simulink model "Comparator"  (R2015a)
settings: Solver=ode23t  StartTime=0.0  StopTime=10.0  RelTol=1e-10
libraries: fl_lib x29, nesl_utility x9, elec_lib x6, pe_lib x1, powerlib x1
settings Model: Creator=saifur  LastModifiedBy=saifur

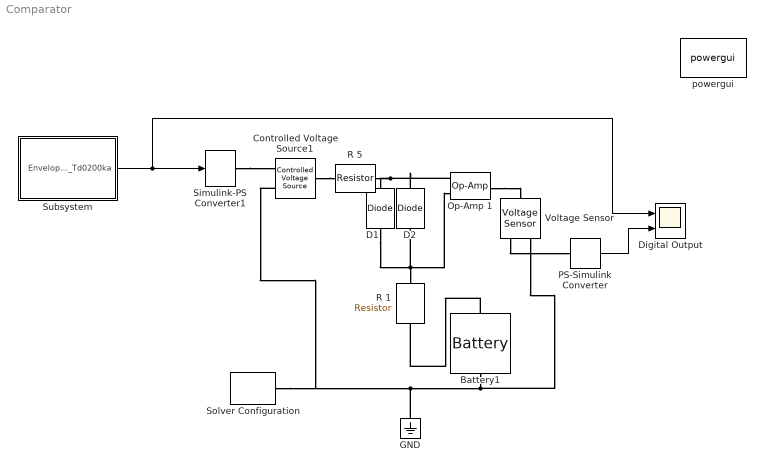
== system Comparator ==
  Battery1 : pe_lib/Sources/Battery  Vnom=6 V  AH=50 hr*A  AH0=50 hr*A  V1=0.5 V  AH1=25 hr*A  R1=2 Ohm  R2=inf Ohm  alpha=1  beta=1  G2=0 S
  Controlled Voltage Source1 : fl_lib/Electrical/Electrical Sources/Controlled Voltage Source
  D1 : fl_lib/Electrical/Electrical Elements/Diode  Vf=0.6 V  Ron=0.3 Ohm  Goff=1e-8 1/Ohm  i_specify=off  i_priority=High  i=0 A  v_specify=off  v_priority=High  v=0 V
  D2 : fl_lib/Electrical/Electrical Elements/Diode  Vf=0.6 V  Ron=0.3 Ohm  Goff=1e-8 1/Ohm  i_specify=off  i_priority=High  i=0 A  v_specify=off  v_priority=High  v=0 V
  Digital Output : Scope  NumInputPorts=2
      settings: TimeRange=10  YMin=-1~-1  YMax=1~1
  GND : fl_lib/Electrical/Electrical Elements/Electrical Reference
  Op-Amp 1 : fl_lib/Electrical/Electrical Elements/Op-Amp  outI_specify=off  outI_priority=High  outI=0 A
  PS-Simulink Converter : nesl_utility/PS-Simulink Converter  PhysicalDomain=network_engine_domain  SubClassName=ps_output  LeftPortType=input  RightPortType=output  PseudoPeriodic=off  Frequencies=[]  Unit=1  AffineConversion=off
  R 1 : elec_lib/Passive Devices/Resistor  R=2.154 kOhm  noise_mode=0  Tdevice=25 C  sample_time=0.001 s  repeatability=1  auto_seed=418932850  user_seed=0
  R 5 : elec_lib/Passive Devices/Resistor  R=2.5 kOhm  noise_mode=0  Tdevice=25 C  sample_time=0.001 s  repeatability=1  auto_seed=2715962282  user_seed=0
  Simulink-PS Converter1 : nesl_utility/Simulink-PS Converter  PhysicalDomain=network_engine_domain  SubClassName=ps_input  LeftPortType=input  RightPortType=output  PseudoPeriodic=off  Frequencies=[]  NoiseDistribution=none  NoiseParameters=[]  Unit=V  AffineConversion=off  InputFiltering=off  SimscapeFilterOrder=1  InputFilterTimeConstant=0.001  UdotUserProvided=1
  Solver Configuration : nesl_utility/Solver Configuration  PhysicalDomain=network_engine_domain  SubClassName=solver  LeftPortType=input  RightPortType=generic  Accelerate=off  Tones=[]  Harmonics=[]  SimulateNoise=off  Profile=off  UseLocalSampling=off  EnableSwitchedLinearOptims=on  FrequencyDomain=off  UseCCode=off  RelTol=0.001  AbsTol=1e-06  MinStep=1e-09  ToWorkspace=off  RevertToSquareIcSolve=off  NumHomotopyIterations=100  DoDC=on  ResidualTolerance=1e-09  UseLocalSolver=off  LocalSolverChoice=NE_BACKWARD_EULER_ADVANCER  LocalSolverSampleTime=0.001  DoFixedCost=off  MaxNonlinIter=3  MaxModeIter=2  LinearAlgebra=Sparse  DelaysMemoryBudget=1024  AutomaticFiltering=on  FilteringTimeConstant=0.001
  Subsystem : Subsystem
  Voltage Sensor : fl_lib/Electrical/Electrical Sensors/Voltage Sensor
  powergui : powerlib/powergui  Priority=1  SimulationMode=Continuous  SolverType=Tustin/Backward Euler (TBE)  SampleTime=50e-6  frequency=60  SPID=on  DisableSnubberDevices=off  DisableRonSwitches=off  DisableVfSwitches=off  SwTol=0  DisplayEquations=on  Interpol=off  methode=off  Ts=100  FunctionMessages=off  echomessages=off  HookPort=off  EnableUseOfTLC=off  x0status=blocks  frequencyindice=0  Pbase=100e6  ErrMax=1e-4  Iterations=50  UnitsV=kV  UnitsW=MW  buscounter=0  RestoreLinks=warning  ResistiveCurrentMeasurement=off  Frange=[0:2:500]  Ylog=off  Xlog=on  ShowGrid=off  save=off  variable=ZData  structure=0  ZoomFFT=off  StartTime=0.0  cycles=1  DisplayStyle=1  fundamental=60  FreqAxis=off  MaxFrequency=1000  frequencyindicesteady=1  RmsSteady=1  display=off
  wires:
  PS-Simulink Converter/1 -> Digital Output/2
  Subsystem/1("Envelope_Td0200ka ") -> Digital Output/1, Simulink-PS Converter1/1
  connections:
  Simulink-PS Converter1/RConn1 -- Controlled Voltage Source1/RConn1
  Controlled Voltage Source1/LConn1 -- R 5/RConn1
  Voltage Sensor/RConn1 -- PS-Simulink Converter/LConn1
  R 5/LConn1 -- Op-Amp 1/LConn1 -- D2/LConn1 -- D1/RConn1
  D1/LConn1 -- R 1/RConn1 -- D2/RConn1 -- Op-Amp 1/LConn2
  Battery1/LConn1 -- R 1/LConn1
  Controlled Voltage Source1/RConn2 -- Solver Configuration/RConn1 -- Voltage Sensor/RConn2 -- Battery1/RConn1 -- GND/LConn1
  Op-Amp 1/RConn1 -- Voltage Sensor/LConn1

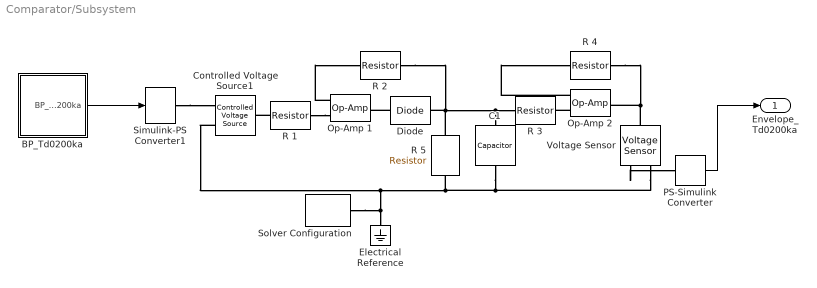
== system Comparator/Subsystem ==
  BP_Td0200ka : Subsystem
  C1 : fl_lib/Electrical/Electrical Elements/Capacitor  c=1e-6 F  r=1e-6 Ohm  g=0 1/Ohm  i_specify=off  i_priority=High  i=0 A  v_specify=off  v_priority=High  v=0 V  vc_specify=off  vc_priority=High  vc=0 V
  Controlled Voltage Source1 : fl_lib/Electrical/Electrical Sources/Controlled Voltage Source
  Diode : fl_lib/Electrical/Electrical Elements/Diode  Vf=0.6 V  Ron=0.3 Ohm  Goff=1e-8 1/Ohm  i_specify=off  i_priority=High  i=0 A  v_specify=off  v_priority=High  v=0 V
  Electrical Reference : fl_lib/Electrical/Electrical Elements/Electrical Reference
  Op-Amp 1 : fl_lib/Electrical/Electrical Elements/Op-Amp  outI_specify=off  outI_priority=High  outI=0 A
  Op-Amp 2 : fl_lib/Electrical/Electrical Elements/Op-Amp  outI_specify=off  outI_priority=High  outI=0 A
  PS-Simulink Converter : nesl_utility/PS-Simulink Converter  PhysicalDomain=network_engine_domain  SubClassName=ps_output  LeftPortType=input  RightPortType=output  PseudoPeriodic=off  Frequencies=[]  Unit=1  AffineConversion=off
  R 1 : fl_lib/Electrical/Electrical Elements/Resistor  R=1 Ohm  i_specify=off  i_priority=High  i=0 A  v_specify=off  v_priority=High  v=0 V
  R 2 : elec_lib/Passive Devices/Resistor  R=1 Ohm  noise_mode=0  Tdevice=25 C  sample_time=0.001 s  repeatability=1  auto_seed=3546856910  user_seed=0
  R 3 : elec_lib/Passive Devices/Resistor  R=1 Ohm  noise_mode=0  Tdevice=25 C  sample_time=0.001 s  repeatability=1  auto_seed=2312163153  user_seed=0
  R 4 : elec_lib/Passive Devices/Resistor  R=1 Ohm  noise_mode=0  Tdevice=25 C  sample_time=0.001 s  repeatability=1  auto_seed=4278366030  user_seed=0
  R 5 : elec_lib/Passive Devices/Resistor  R=1 Ohm  noise_mode=0  Tdevice=25 C  sample_time=0.001 s  repeatability=1  auto_seed=335761340  user_seed=0
  Simulink-PS Converter1 : nesl_utility/Simulink-PS Converter  PhysicalDomain=network_engine_domain  SubClassName=ps_input  LeftPortType=input  RightPortType=output  PseudoPeriodic=off  Frequencies=[]  NoiseDistribution=none  NoiseParameters=[]  Unit=V  AffineConversion=off  InputFiltering=off  SimscapeFilterOrder=1  InputFilterTimeConstant=0.001  UdotUserProvided=1
  Solver Configuration : nesl_utility/Solver Configuration  PhysicalDomain=network_engine_domain  SubClassName=solver  LeftPortType=input  RightPortType=generic  Accelerate=off  Tones=[]  Harmonics=[]  SimulateNoise=off  Profile=off  UseLocalSampling=off  EnableSwitchedLinearOptims=on  FrequencyDomain=off  UseCCode=off  RelTol=0.001  AbsTol=1e-06  MinStep=1e-09  ToWorkspace=off  RevertToSquareIcSolve=off  NumHomotopyIterations=100  DoDC=on  ResidualTolerance=1e-09  UseLocalSolver=off  LocalSolverChoice=NE_BACKWARD_EULER_ADVANCER  LocalSolverSampleTime=0.001  DoFixedCost=off  MaxNonlinIter=3  MaxModeIter=2  LinearAlgebra=Sparse  DelaysMemoryBudget=1024  AutomaticFiltering=on  FilteringTimeConstant=0.001
  Voltage Sensor : fl_lib/Electrical/Electrical Sensors/Voltage Sensor
  "Envelope_Td0200ka " : Outport
  wires:
  BP_Td0200ka/1(BP_Td0200ka) -> Simulink-PS Converter1/1
  PS-Simulink Converter/1 -> "Envelope_Td0200ka "/1
  connections:
  Simulink-PS Converter1/RConn1 -- Controlled Voltage Source1/RConn1
  R 1/RConn1 -- Op-Amp 1/LConn1
  R 2/RConn1 -- R 3/LConn1 -- C1/LConn1 -- R 5/LConn1 -- Diode/RConn1
  Op-Amp 2/LConn2 -- R 4/LConn1
  Voltage Sensor/RConn1 -- PS-Simulink Converter/LConn1
  C1/RConn1 -- Voltage Sensor/RConn2 -- Solver Configuration/RConn1 -- Electrical Reference/LConn1 -- Controlled Voltage Source1/RConn2 -- R 5/RConn1
  R 4/RConn1 -- Voltage Sensor/LConn1 -- Op-Amp 2/RConn1
  R 1/LConn1 -- Controlled Voltage Source1/LConn1
  Diode/LConn1 -- Op-Amp 1/RConn1
  Op-Amp 1/LConn2 -- R 2/LConn1
  Op-Amp 2/LConn1 -- R 3/RConn1

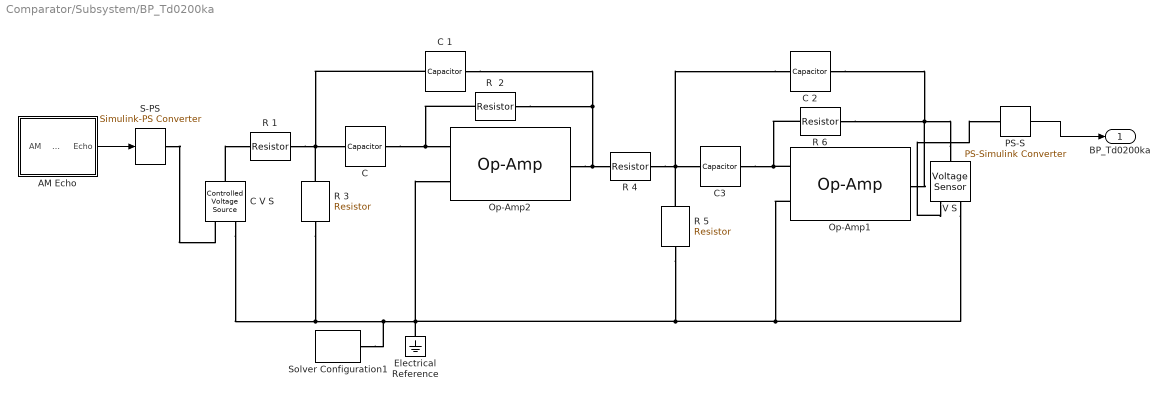
== system Comparator/Subsystem/BP_Td0200ka ==
  AM Echo : Subsystem
  C : fl_lib/Electrical/Electrical Elements/Capacitor  c=10 nF  r=1e-6 Ohm  g=0 1/Ohm  i_specify=off  i_priority=High  i=0 A  v_specify=off  v_priority=High  v=0 V  vc_specify=off  vc_priority=High  vc=0 V
  "C 1 " : fl_lib/Electrical/Electrical Elements/Capacitor  c=1e-6 F  r=1e-6 Ohm  g=0 1/Ohm  i_specify=off  i_priority=High  i=0 A  v_specify=off  v_priority=High  v=0 V  vc_specify=off  vc_priority=High  vc=0 V
  C 2 : fl_lib/Electrical/Electrical Elements/Capacitor  c=1e-6 F  r=1e-6 Ohm  g=0 1/Ohm  i_specify=off  i_priority=High  i=0 A  v_specify=off  v_priority=High  v=0 V  vc_specify=off  vc_priority=High  vc=0 V
  C V S : fl_lib/Electrical/Electrical Sources/Controlled Voltage Source
  C3 : fl_lib/Electrical/Electrical Elements/Capacitor  c=10 nF  r=1e-6 Ohm  g=0 1/Ohm  i_specify=off  i_priority=High  i=0 A  v_specify=off  v_priority=High  v=0 V  vc_specify=off  vc_priority=High  vc=0 V
  Electrical Reference : fl_lib/Electrical/Electrical Elements/Electrical Reference
  Op-Amp1 : fl_lib/Electrical/Electrical Elements/Op-Amp  outI_specify=off  outI_priority=High  outI=0 A
  Op-Amp2 : fl_lib/Electrical/Electrical Elements/Op-Amp  outI_specify=off  outI_priority=High  outI=0 A
  PS-S : nesl_utility/PS-Simulink Converter  PhysicalDomain=network_engine_domain  SubClassName=ps_output  LeftPortType=input  RightPortType=output  PseudoPeriodic=off  Frequencies=[]  Unit=1  AffineConversion=off
  R  2 : fl_lib/Electrical/Electrical Elements/Resistor  R=4.73 kOhm  i_specify=off  i_priority=High  i=0 A  v_specify=off  v_priority=High  v=0 V
  R 1 : fl_lib/Electrical/Electrical Elements/Resistor  R=519.8 Ohm  i_specify=off  i_priority=High  i=0 A  v_specify=off  v_priority=High  v=0 V
  R 3 : fl_lib/Electrical/Electrical Elements/Resistor  R=0.91 Ohm  i_specify=off  i_priority=High  i=0 A  v_specify=off  v_priority=High  v=0 V
  R 4 : fl_lib/Electrical/Electrical Elements/Resistor  R=763.73 Ohm  i_specify=off  i_priority=High  i=0 A  v_specify=off  v_priority=High  v=0 V
  R 5 : fl_lib/Electrical/Electrical Elements/Resistor  R=1.34 kOhm  i_specify=off  i_priority=High  i=0 A  v_specify=off  v_priority=High  v=0 V
  R 6 : fl_lib/Electrical/Electrical Elements/Resistor  R=6.95 kOhm  i_specify=off  i_priority=High  i=0 A  v_specify=off  v_priority=High  v=0 V
  S-PS : nesl_utility/Simulink-PS Converter  PhysicalDomain=network_engine_domain  SubClassName=ps_input  LeftPortType=input  RightPortType=output  PseudoPeriodic=off  Frequencies=[]  NoiseDistribution=none  NoiseParameters=[]  Unit=V  AffineConversion=off  InputFiltering=off  SimscapeFilterOrder=1  InputFilterTimeConstant=0.001  UdotUserProvided=1
  Solver Configuration1 : nesl_utility/Solver Configuration  PhysicalDomain=network_engine_domain  SubClassName=solver  LeftPortType=input  RightPortType=generic  Accelerate=off  Tones=[]  Harmonics=[]  SimulateNoise=off  Profile=off  UseLocalSampling=off  EnableSwitchedLinearOptims=on  FrequencyDomain=off  UseCCode=off  RelTol=0.001  AbsTol=1e-06  MinStep=1e-09  ToWorkspace=off  RevertToSquareIcSolve=off  NumHomotopyIterations=100  DoDC=on  ResidualTolerance=1e-09  UseLocalSolver=off  LocalSolverChoice=NE_BACKWARD_EULER_ADVANCER  LocalSolverSampleTime=0.001  DoFixedCost=off  MaxNonlinIter=3  MaxModeIter=2  LinearAlgebra=Sparse  DelaysMemoryBudget=1024  AutomaticFiltering=on  FilteringTimeConstant=0.001
  V S : fl_lib/Electrical/Electrical Sensors/Voltage Sensor
  BP_Td0200ka : Outport
  wires:
  AM Echo/1("AM           Echo ") -> S-PS/1
  PS-S/1 -> BP_Td0200ka/1
  connections:
  C V S/LConn1 -- R 1/RConn1
  C/RConn1 -- R  2/RConn1 -- Op-Amp2/LConn2
  C3/RConn1 -- R 6/LConn1 -- Op-Amp1/LConn1
  V S/LConn1 -- C 2/RConn1 -- R 6/RConn1 -- Op-Amp1/RConn1
  R 5/RConn1 -- C V S/RConn2 -- R 3/RConn1 -- Solver Configuration1/RConn1 -- Op-Amp2/LConn1 -- Electrical Reference/LConn1 -- V S/RConn2 -- Op-Amp1/LConn2
  C 2/LConn1 -- R 4/RConn1 -- R 5/LConn1 -- C3/LConn1
  "C 1 "/LConn1 -- R 1/LConn1 -- R 3/LConn1 -- C/LConn1
  Op-Amp2/RConn1 -- R  2/LConn1 -- "C 1 "/RConn1 -- R 4/LConn1
  V S/RConn1 -- PS-S/LConn1
  S-PS/RConn1 -- C V S/RConn1

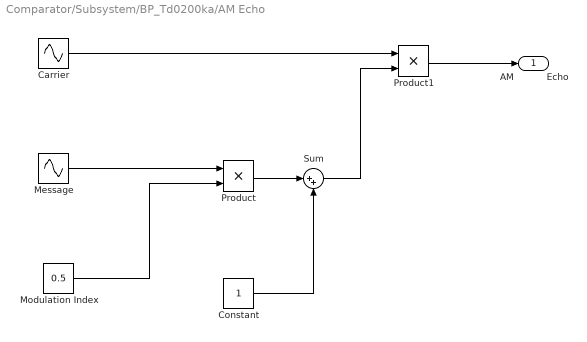
== system Comparator/Subsystem/BP_Td0200ka/AM Echo ==
  Carrier : Sin  Frequency=2*pi*25  SampleTime=1/5000
  Constant : Constant
  Message : Sin  Amplitude=5  Frequency=2*pi*100  SampleTime=1/5000
  Modulation Index : Constant  Value=0.5
  Product : Product
  Product1 : Product
  Sum : Sum  Inputs=|++
  "AM           Echo " : Outport
  wires:
  Product/1 -> Sum/1
  Modulation Index/1 -> Product/2
  Message/1 -> Product/1
  Constant/1 -> Sum/2
  Carrier/1 -> Product1/1
  Sum/1 -> Product1/2
  Product1/1 -> "AM           Echo "/1
